simulink subsystem "ac"  (R2022a)
settings: Solver=VariableStepAuto  StartTime=0.0  StopTime=10.0  RelTol=1e-3
libraries: fl_lib x1, nesl_utility x1
settings Model: Creator=Cristobal  LastModifiedBy=Cristobal

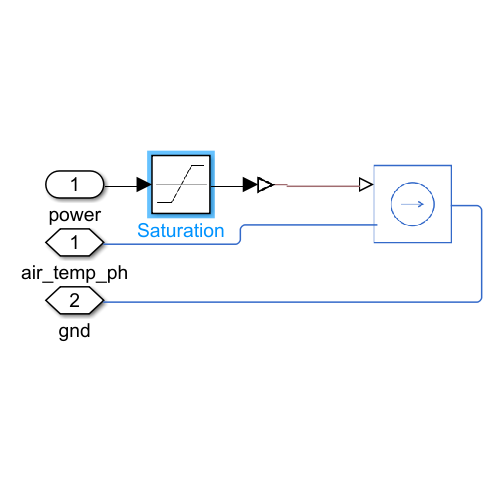
[thumbnail: Simulink's stored preview of the top-level diagram]
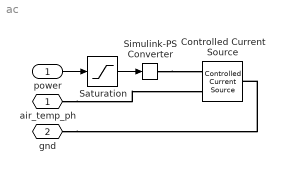
== system ac ==
  power : Inport
  Controlled Current Source : fl_lib/Electrical/Electrical Sources/Controlled Current Source
      settings: SourceProductBaseCode=PW,SS,VE
  Saturation : Saturate  UpperLimit=+inf  LowerLimit=0
  Simulink-PS Converter : nesl_utility/Simulink-PS Converter  PhysicalDomain=network_engine_domain  SubClassName=ps_input  LeftPortType=input  RightPortType=output  PseudoPeriodic=off  Frequencies=[]  NoiseDistribution=none  NoiseParameters=[]  Unit=1  AffineConversion=off  FilteringAndDerivatives=provide  SimscapeFilterOrder=1  InputFilterTimeConstant=0.001  UdotUserProvided=0
      settings: SourceProductBaseCode=SS,PW,VE
  air_temp_ph : PMIOPort  Side=Left
  gnd : PMIOPort  Port=2  Side=Left
  wires:
  power/1 -> Saturation/1
  Saturation/1 -> Simulink-PS Converter/1
  connections:
  Simulink-PS Converter/RConn1 -- Controlled Current Source/RConn1
  air_temp_ph/RConn1 -- Controlled Current Source/RConn2
  gnd/RConn1 -- Controlled Current Source/LConn1
